simulink model "Simulation3"  (R2023b)
settings: Solver=VariableStepAuto  StartTime=0.0  StopTime=2  RelTol=1e-3
settings Model: Creator=vande_2  LastModifiedBy=vande_2

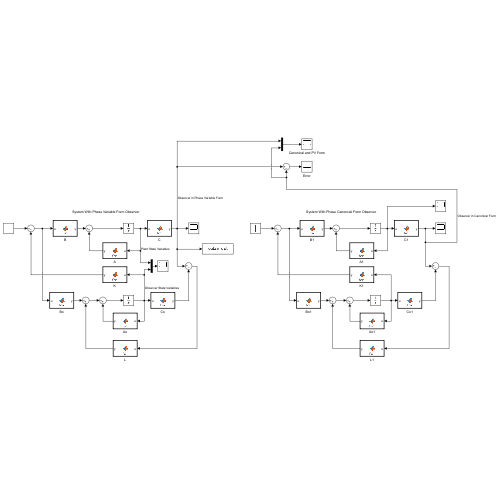
[thumbnail: Simulink's stored preview of the top-level diagram]
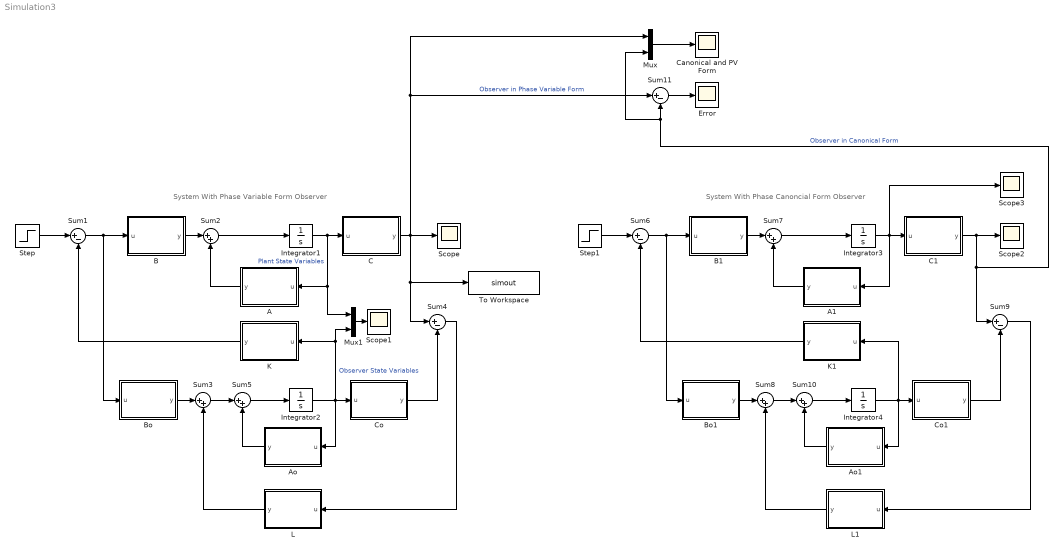
== system Simulation3 ==
  note: System With Phase Variable Form Observer
  note: System With Phase Canoncial Form Observer
  A : MATLAB Function  TreatAsAtomicUnit=on
  A1 : MATLAB Function  TreatAsAtomicUnit=on
  Ao : MATLAB Function  TreatAsAtomicUnit=on
  Ao1 : MATLAB Function  TreatAsAtomicUnit=on
  B : MATLAB Function  TreatAsAtomicUnit=on
  B1 : MATLAB Function  TreatAsAtomicUnit=on
  Bo : MATLAB Function  TreatAsAtomicUnit=on
  Bo1 : MATLAB Function  TreatAsAtomicUnit=on
  C : MATLAB Function  TreatAsAtomicUnit=on
  C1 : MATLAB Function  TreatAsAtomicUnit=on
  Canonical and PV Form : Scope
  Co : MATLAB Function  TreatAsAtomicUnit=on
  Co1 : MATLAB Function  TreatAsAtomicUnit=on
  Error : Scope
  Integrator1 : Integrator
  Integrator2 : Integrator  InitialCondition=[2;2]
  Integrator3 : Integrator
  Integrator4 : Integrator  InitialCondition=[2;2]
  K : MATLAB Function  TreatAsAtomicUnit=on
  K1 : MATLAB Function  TreatAsAtomicUnit=on
  L : MATLAB Function  TreatAsAtomicUnit=on
  L1 : MATLAB Function  TreatAsAtomicUnit=on
  Mux : Mux  Inputs=2
  Mux1 : Mux  Inputs=2
  Scope{,1..3} (4 alike) : Scope
  Step : Step  Time=0  SampleTime=0
  Step1 : Step  Time=0  SampleTime=0
  Sum{1,4,6,9,11} (5 alike) : Sum  Inputs=|+-
  Sum{2..3,5,7..8,10} (6 alike) : Sum  Inputs=|++
  To Workspace : ToWorkspace  VariableName=simout  SaveFormat=Timeseries  SampleTime=-1
  wires:
  B/1(y) -> Sum2/1
  Integrator2/1 -> Ao/1(u), Mux1/2, K/1(u), Co/1(u)  "Observer State Variables"
  Sum5/1 -> Integrator2/1
  A/1(y) -> Sum2/2
  K/1(y) -> Sum1/2
  Sum1/1 -> B/1(u), Bo/1(u)
  Co/1(y) -> Sum4/2
  Integrator1/1 -> Mux1/1, A/1(u), C/1(u)  "Plant State Variables"
  Step/1 -> Sum1/1
  Sum2/1 -> Integrator1/1
  Bo/1(y) -> Sum3/1
  Ao/1(y) -> Sum5/2
  C/1(y) -> Sum4/1, To Workspace/1, Sum11/1, Mux/1, Scope/1  "Observer in Phase Variable Form"
  Sum3/1 -> Sum5/1
  Sum4/1 -> L/1(u)
  L/1(y) -> Sum3/2
  Sum6/1 -> B1/1(u), Bo1/1(u)
  Sum8/1 -> Sum10/1
  Sum9/1 -> L1/1(u)
  L1/1(y) -> Sum8/2
  Integrator4/1 -> Ao1/1(u), K1/1(u), Co1/1(u)
  Sum10/1 -> Integrator4/1
  Bo1/1(y) -> Sum8/1
  K1/1(y) -> Sum6/2
  B1/1(y) -> Sum7/1
  Integrator3/1 -> Scope3/1, C1/1(u), A1/1(u)
  A1/1(y) -> Sum7/2
  Co1/1(y) -> Sum9/2
  Step1/1 -> Sum6/1
  C1/1(y) -> Mux/2, Sum11/2, Sum9/1, Scope2/1  "Observer in Canonical Form"
  Ao1/1(y) -> Sum10/2
  Sum7/1 -> Integrator3/1
  Mux/1 -> Canonical and PV Form/1
  Sum11/1 -> Error/1
  Mux1/1 -> Scope1/1

== matlab function Simulation3/K1 ==
  data: u input; y output
function y = fcn(u)
K = [98.1690 7.4031];
y = K*u;

== matlab function Simulation3/L1 ==
  data: u input; y output
function y = fcn(u)
L = [1012.755;  125174.327];
y = L*u;

== matlab function Simulation3/A ==
  data: u input; y output
function y = fcn(u)
A = [0 1; 0 -0.5696];
y = A*u;

== matlab function Simulation3/Bo ==
  data: u input; y output
function y = fcn(u)
B = [0; 1];
y = B*u;

== matlab function Simulation3/Co ==
  data: u input; y output
function y = fcn(u)
C = [0.0784, 0];
y = C*u;

== matlab function Simulation3/B ==
  data: u input; y output
function y = fcn(u)
B = [0; 1];
y = B*u;

== matlab function Simulation3/C ==
  data: u input; y output
function y = fcn(u)
C = [0.07843, 0];
y = C*u;

== matlab function Simulation3/L ==
  data: u input; y output
function y = fcn(u)
L = [1012.755;  125174.327];
y = L*u;

== matlab function Simulation3/K ==
  data: u input; y output
function y = fcn(u)
K = [98.1690 7.4031];
y = K*u;

== matlab function Simulation3/A1 ==
  data: u input; y output
function y = fcn(u)
A = [0 1; 0 -0.5696];
y = A*u;

== matlab function Simulation3/Ao ==
  data: u input; y output
function y = fcn(u)
A = [0 1; 0 -0.5696];
y = A*u;

== matlab function Simulation3/Ao1 ==
  data: u input; y output
function y = fcn(u)
A = [-0.5696 1; 0 0];
y = A*u;

== matlab function Simulation3/B1 ==
  data: u input; y output
function y = fcn(u)
B = [0; 1];
y = B*u;

== matlab function Simulation3/Bo1 ==
  data: u input; y output
function y = fcn(u)
B = [0; 0.0784];
y = B*u;

== matlab function Simulation3/C1 ==
  data: u input; y output
function y = fcn(u)
C = [0.07843, 0];
y = C*u;

== matlab function Simulation3/Co1 ==
  data: u input; y output
function y = fcn(u)
C = [1, 0];
y = C*u;
